simulink model "Control_BA"  (R2023b)
settings: Solver=VariableStepAuto  StartTime=0.0  StopTime=10.0  RelTol=1e-3
settings Model: Creator=Alberto  LastModifiedBy=Alberto

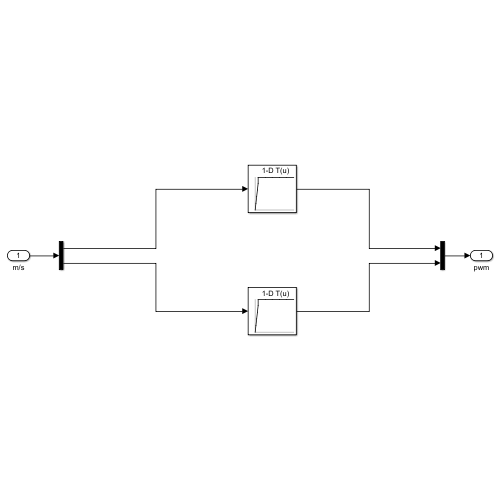
[thumbnail: Simulink's stored preview of the top-level diagram]
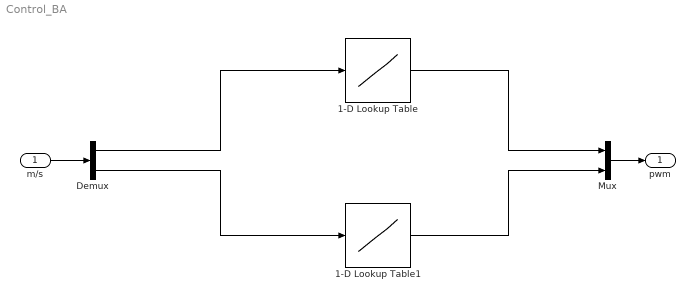
== system Control_BA ==
  m/s : Inport
  1-D Lookup Table : Lookup_n-D  NumberOfTableDimensions=1  BreakpointsForDimension1=[-0.461627960205078 -0.384681701660156 -0.2821044921875 -0.179512023925781 -0.0769424438476563 0 1 2 3 4 5]  Table=[-255 -201 -150 -100 -50 0 0.761594155955765 0.964027580075817 0.99505475368673 0.999329299739067 0.999909204262595]  InternalRulePriority=Speed  RndMeth=Simplest
  1-D Lookup Table1 : Lookup_n-D  NumberOfTableDimensions=1  BreakpointsForDimension1=[-0.461627960205078 -0.384681701660156 -0.2821044921875 -0.179512023925781 -0.0769424438476563 0 1 2 3 4 5]  Table=[-255 -201 -150 -100 -50 0 0.761594155955765 0.964027580075817 0.99505475368673 0.999329299739067 0.999909204262595]  InternalRulePriority=Speed  RndMeth=Simplest
  Demux : Demux  Outputs=2
  Mux : Mux  Inputs=2
  pwm : Outport
  wires:
  Mux/1 -> pwm/1
  1-D Lookup Table/1 -> Mux/1
  m/s/1 -> Demux/1
  Demux/1 -> 1-D Lookup Table/1
  Demux/2 -> 1-D Lookup Table1/1
  1-D Lookup Table1/1 -> Mux/2
